simulink model "uav_simple_flight_model"  (R2024a)
settings: Solver=VariableStepAuto  StartTime=0.0  StopTime=10.0  RelTol=1e-3
libraries: visionsinks x1, sim3dcameralib x1, sim3dlib x1, uavsim3dlib x1
settings Model: Creator=The MathWorks, Inc.  LastModifiedBy=The MathWorks, Inc.
settings SolverCC: AlgebraicLoopSolver=TrustRegion
settings DebuggingCC: UnconnectedInputMsg=warning  UnconnectedOutputMsg=warning  UnconnectedLineMsg=warning
settings ModelReferenceCC: EnableRefExpFcnMdlSchedulingChecks=on
settings RTWCC: GPUComputeCapability=3.5  DLArmComputeVersion=19.05

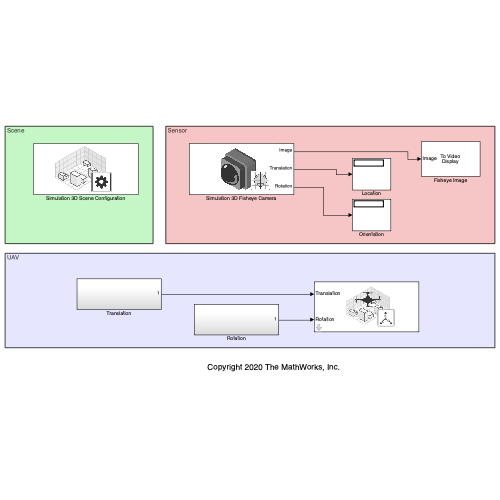
[thumbnail: Simulink's stored preview of the top-level diagram]
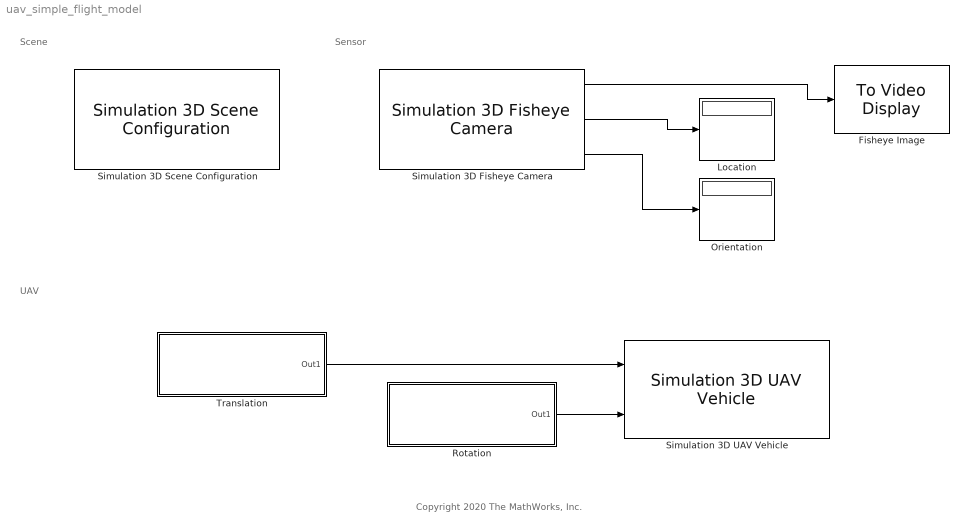
== system uav_simple_flight_model ==
  note: UAV
  note: Sensor
  note: Scene
  note: Copyright 2020 The MathWorks, Inc.
  Fisheye Image : visionsinks/To Video Display  windowSizeMode=Normal  openAtMdlStart=on  fullScreen=off  videoWindowX=536805376  videoWindowY=536805376  saveWindowSize=off  videoWindowWidth=640  videoWindowHeight=640  inputColorFormat=RGB  inputType=Obsolete  imagePorts=One multidimensional signal  OutputDevice=On-screen video monitor  dataOrg=Column-major  isWindowOpen=off
  Location : Display
  Orientation : Display
  Rotation : Subsystem
  Simulation 3D Fisheye Camera : sim3dcameralib/Simulation 3D Fisheye Camera  Priority=1  sensorTag=Sim3dSensor1  sensorId=1  sensorName=Sim3dSensor1  vehTagList={'Quadrotor1';'Scene Origin'}  vehTag=Quadrotor1  mountLoc=Origin  offsetFlag=on  tmountOffset=[0.1, 0, 0]  extTmount=off  rmountOffset=[0, 0, 0]  extRmount=off  OpticalCenter=[640, 360]  ImageSize=[720, 1280]  RadialDistortion=[320, -0.0005, 0, 0]  StretchMatrix=[1, 0; 0, 1]  TransformOutportEnabled=on  SampleTime=-1  mountPoint=[0.1 0 0]  mountOrientation=[0 0 0]  aMode=4  ID=1
      settings: LibrarySourceBlock=uavsim3dlib/Simulation 3D Fisheye Camera
  Simulation 3D Scene Configuration : sim3dlib/Simulation 3D Scene Configuration  Priority=0  ProjectFormat=Default Scenes  SceneDesc=US city block  ProjectName=/System/Volumes/Data/mathworks/devel/bat/filer/batfs1904-0/Bdoc24a.2528353/build/matlab/toolbox/shared/sim3d_projects/automotive_project_mac/UE/MacNoEditor/AutoVrtlEnv.sh  ScenePath=/Game/Maps/USCityBlock  EnableOpenDRIVE=off  vehTagList={'Quadrotor1';'Scene Origin'}  vehTag=Scene Origin  FreeCameraInitialTranslation=[0, 0, 0]  FreeCameraDefaultInitialTranslation=[-6, 0, 2]  FreeCameraInitialRotation=[0, 0, 0]  FreeCameraDefaultInitialRotation=[0, -15, 0]  OpVisEn=off  Ts=1/60  EnableWindow=on  EnableRemoteAccess=off  EnableWeather=off  SunAzimuth=90  SunAltitude=40.0  EnableGeospatialSun=off  Latitude=0  Longitude=0  Date=2023-01-01  Time=10:30:00  GeoTimeZone=-5.0  SunDaylightSaving=off  wind=1  clouds=10  EnableVolumetricClouds=off  CloudCoverage=0  CloudAltitude=6  fog=0  rain=0  RaindropsEffect=off  SnowDensity=0  EnableGeospatial=off  UseTrueOrigin=off  OriginHeight=200  OriginLatitude=40.744652  OriginLongitude=-73.988864  MapStyle=Aerial  AdditionalAssetIDs=[]  UseAdvancedSunSky=off  SolarTime=11  TimeZone=-5  Day=21  Month=9  Year=2022  UseDaylightSavingTime=on  DSTStartDay=10  DSTStartMonth=3  DSTEndDay=3  DSTEndMonth=11  DSTSwitchHour=2  sensorTag=MainCamera1  sensorId=1  sensorName=MainCamera1  mountLoc=Origin  offsetFlag=off  tmountOffset=[0, 0, 0]  rmountOffset=[0, 0, 0]  HorizontalResolution=1280  VerticalResolution=720  HorizontalFOV=60  mountPoint=[0 0 0]  mountOrientation=[0 0 0]  aMode=4  ID=1  GeoTrigger=Inactive
      settings: LibrarySourceBlock=uavsim3dlib/Simulation 3D Scene Configuration
  Simulation 3D UAV Vehicle : uavsim3dlib/Simulation 3D UAV Vehicle  Mesh=Quadrotor  MeshPath=/MathWorksUAVContent/UAVs/HexaRotorUAV/HexaRotor.HexaRotor  Color=Black  ActorName=Quadrotor1  UseGlobalFrame=off  InitialTranslation=[0 5 1.5]  InitialRotation=[0 0 0]  InitialTranslationGlobal=[0 0 0]  InitialGeoOrigin=[0 0 0]  InitialRotationGlobal=[0 0 0]  SampleTime=-1  ActorType=SimulinkVehicle  ID=C  aMode=4  ActorTag=Quadrotor1
  Translation : Subsystem
  wires:
  Translation/1(Out1) -> Simulation 3D UAV Vehicle/1
  Rotation/1(Out1) -> Simulation 3D UAV Vehicle/2
  Simulation 3D Fisheye Camera/2 -> Location/1
  Simulation 3D Fisheye Camera/3 -> Orientation/1
  Simulation 3D Fisheye Camera/1 -> Fisheye Image/1

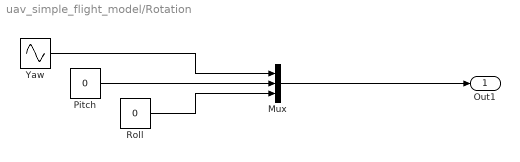
== system uav_simple_flight_model/Rotation ==
  Mux : Mux  Inputs=3
  Pitch : Constant  Value=0
  Roll : Constant  Value=0
  Yaw : Sin  SampleTime=0
  Out1 : Outport
  wires:
  Pitch/1 -> Mux/2
  Roll/1 -> Mux/3
  Yaw/1 -> Mux/1
  Mux/1 -> Out1/1

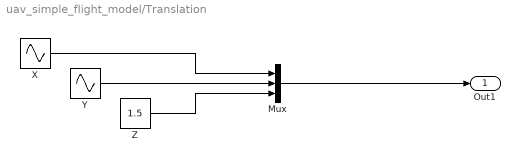
== system uav_simple_flight_model/Translation ==
  Mux : Mux  Inputs=3
  X : Sin  Amplitude=5  Frequency=2*pi/10  SampleTime=0
  Y : Sin  Amplitude=5  Frequency=2*pi/10  Phase=pi/2  SampleTime=0
  Z : Constant  Value=1.5
  Out1 : Outport
  wires:
  Y/1 -> Mux/2
  Z/1 -> Mux/3
  X/1 -> Mux/1
  Mux/1 -> Out1/1
